simulink model "Modelado_SPWM_Vehiculo"  (R2018a)
settings: Solver=VariableStepAuto  StartTime=0.0  StopTime=1/50  RelTol=1e-3
libraries: powerlib_meascontrol x2
settings Model: Creator=user  LastModifiedBy=user

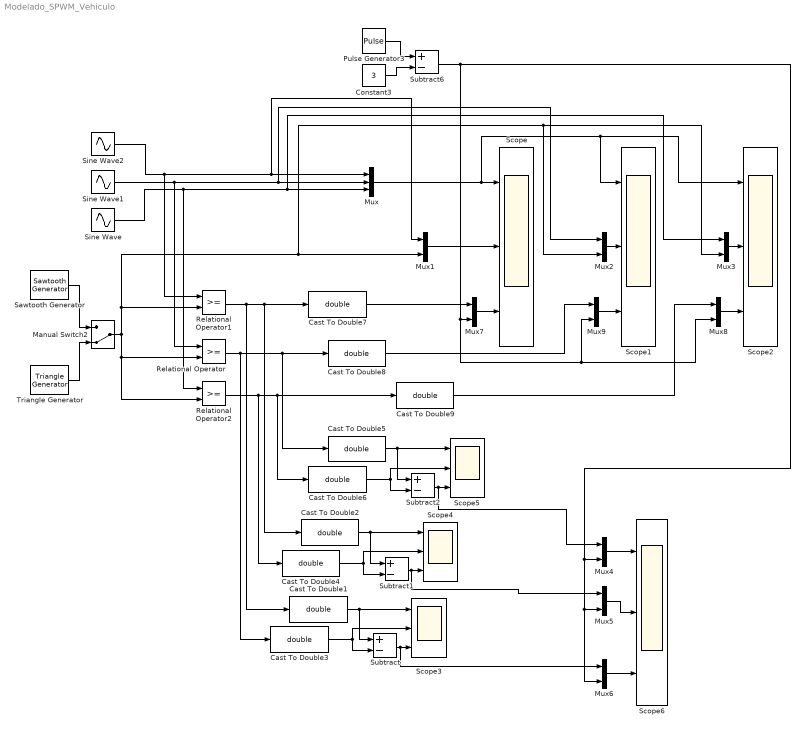
== system Modelado_SPWM_Vehiculo ==
  Cast To Double{1..9} (9 alike) : DataTypeConversion  OutDataTypeStr=double
  Constant3 : Constant  Value=3
  Manual Switch2 : ManualSwitch  CurrentSetting=0
  Mux : Mux  Inputs=3
  Mux{1..9} (9 alike) : Mux  Inputs=2
  Pulse Generator3 : DiscretePulseGenerator  PulseType=Time based  Amplitude=6  Period=1/500  PulseWidth=50  VectorParams1D=off
  Relational Operator : RelationalOperator  OutDataTypeStr=boolean  RndMeth=Simplest
  Relational Operator1 : RelationalOperator  OutDataTypeStr=boolean  RndMeth=Simplest
  Relational Operator2 : RelationalOperator  OutDataTypeStr=boolean  RndMeth=Simplest
  Sawtooth Generator : powerlib_meascontrol/Pulse & Signal Generators/Sawtooth Generator  Freq=1e3  Phase=180  Ts=0
      settings: SourceProductName=Simscape Power Systems
  Scope{,1..6} (7 alike) : Scope  NumInputPorts=3
  Sine Wave : Sin  Frequency=2*pi*50  Phase=4*pi/3  SampleTime=0
  Sine Wave1 : Sin  Frequency=2*pi*50  Phase=2*pi/3  SampleTime=0
  Sine Wave2 : Sin  Frequency=2*pi*50  SampleTime=0
  Subtract{,1..2,6} (4 alike) : Sum  Inputs=+-
  Triangle Generator : powerlib_meascontrol/Pulse & Signal Generators/Triangle Generator  Freq=1e3  Phase=0  Ts=0
  wires:
  Sine Wave/1 -> Relational Operator2/1, Mux3/1, Mux/3
  Mux/1 -> Scope2/1, Scope1/1, Scope/1
  Sine Wave1/1 -> Relational Operator/1, Mux/2, Mux2/1
  Sine Wave2/1 -> Relational Operator1/1, Mux/1, Mux1/1
  Mux1/1 -> Scope/2
  Mux2/1 -> Scope1/2
  Mux3/1 -> Scope2/2
  Relational Operator2/1 -> Cast To Double4/1, Cast To Double6/1, Cast To Double9/1
  Subtract/1 -> Mux6/1, Scope3/3
  Relational Operator/1 -> Cast To Double3/1, Cast To Double5/1, Cast To Double8/1
  Relational Operator1/1 -> Cast To Double1/1, Cast To Double2/1, Cast To Double7/1
  Manual Switch2/1 -> Mux2/2, Mux3/2, Mux1/2, Relational Operator1/2, Relational Operator2/2, Relational Operator/2
  Cast To Double1/1 -> Scope3/1, Subtract/1
  Cast To Double3/1 -> Scope3/2, Subtract/2
  Cast To Double2/1 -> Scope4/1, Subtract1/1
  Cast To Double4/1 -> Scope4/2, Subtract1/2
  Subtract1/1 -> Mux5/1, Scope4/3
  Cast To Double5/1 -> Scope5/1, Subtract2/1
  Cast To Double6/1 -> Scope5/2, Subtract2/2
  Mux4/1 -> Scope6/1
  Mux6/1 -> Scope6/3
  Subtract2/1 -> Mux4/1, Scope5/3
  Mux5/1 -> Scope6/2
  Mux7/1 -> Scope/3
  Cast To Double7/1 -> Mux7/1
  Constant3/1 -> Subtract6/2
  Pulse Generator3/1 -> Subtract6/1
  Subtract6/1 -> Mux4/2, Mux5/2, Mux6/2, Mux7/2, Mux8/2, Mux9/2
  Mux9/1 -> Scope1/3
  Mux8/1 -> Scope2/3
  Cast To Double8/1 -> Mux9/1
  Cast To Double9/1 -> Mux8/1
  Sawtooth Generator/1 -> Manual Switch2/1
  Triangle Generator/1 -> Manual Switch2/2
